simulink model "AnglePWM"  (R2014a)
settings: Solver=FixedStepDiscrete  StartTime=0.0  StopTime=50000  FixedStep=1  RelTol=1e-3
libraries: hdlsllib x1
settings Model: Creator=rogers.a  LastModifiedBy=rogers.a

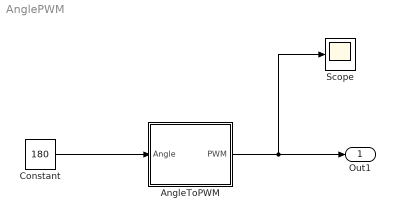
== system AnglePWM ==
  "AngleToPWM " : Subsystem
  Constant : Constant  Value=180  OutDataTypeStr=double
  Scope : Scope
  Out1 : Outport
  wires:
  "AngleToPWM "/1("PWM ") -> Out1/1, Scope/1
  Constant/1 -> "AngleToPWM "/1("Angle ")

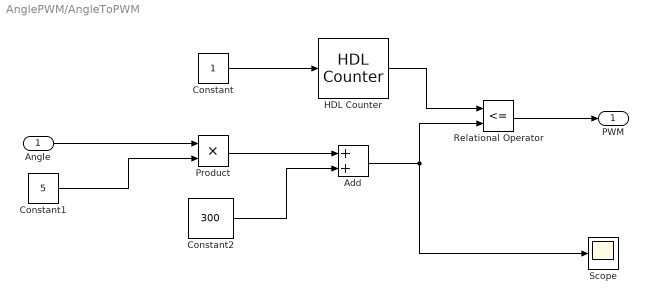
== system AnglePWM/AngleToPWM  ==
  "Angle " : Inport  OutDataTypeStr=double
  Add : Sum
  Constant : Constant  OutDataTypeStr=boolean
  Constant1 : Constant  Value=5  OutDataTypeStr=double
  Constant2 : Constant  Value=300
  HDL Counter : hdlsllib/HDL Operations/HDL Counter  CountType=Count limited  CountInit=0  CountStep=1  CountMax=10000  CountFromType=Initial value  CountFrom=0  CountResetPort=off  CountLoadPort=off  CountEnbPort=on  CountDirPort=off  CountDataType=Unsigned  CountWordLen=32  CountFracLen=0  CountSampTime=1
  Product : Product  SaturateOnIntegerOverflow=on
  Relational Operator : RelationalOperator  Operator=<=  OutDataTypeStr=boolean
  Scope : Scope
  "PWM " : Outport
  wires:
  "Angle "/1 -> Product/1
  Product/1 -> Add/1
  Add/1 -> Relational Operator/2, Scope/1
  Constant1/1 -> Product/2
  Relational Operator/1 -> "PWM "/1
  Constant/1 -> HDL Counter/1
  Constant2/1 -> Add/2
  HDL Counter/1 -> Relational Operator/1
